simulink model "Sim_2025_04_07_Heet"  (R2024b)
settings: Solver=FixedStepAuto  StartTime=0.0  StopTime=2350  FixedStep=0.01  RelTol=1e-3
values from neighbouring files (symbols this model uses):
  cpSn = 230    [Sim_Parameter_Heet.m]
  mB = VB*rohSn    (= 7671.14496)    [Sim_Parameter_Heet.m]
  TU = 35    [Sim_Parameter_Heet.m]
undefined symbols (not defined in the file or in its folder): PLC_1, SIMATIC, UA
libraries: simulink x7, slpidlib x7, opcualib x6
(part 3 of 3)

== matlab function Sim_2025_04_07_Heet/Alte Systeme/Subsystem3/Air knife Betriebszustandsberechnung in Prozent ==
  data: druck1 input; druck2 input; Prozent output
function Prozent  = fcn(druck1, druck2)
%#codegen
% fcn Berechnet die Leistung und den prozentualen Anteil mithilfe einer
%     natürlichen Logarithmusfunktion.
%
% Eingänge:
%   druck1 - Erster Druckwert in mbar
%   druck2 - Zweiter Druckwert in mbar
%
% Ausgänge:
%   Leistung - Berechnete Leistung in Watt
%   Prozent  - Relativer Anteil in Prozent (0% - 100%)
%
% Randbedingungen:
%   - 0 mbar => 0%
%   - 400 mbar => 100%
%   - Dazwischen natürliche Logarithmus-Skalierung

    % Mittelwert berechnen
    druckMittelwert = (druck1 + druck2) / 2;
    
    % Sicherheitsabfragen, um log(0) zu vermeiden
    if druckMittelwert < 20
        druckMittelwert = 0;
    elseif druckMittelwert > 600
        druckMittelwert = 600;
    end

    
    if druckMittelwert == 0
        Prozent = 0;
    else
        Prozent = 100 *druckMittelwert / 600;
    end

    Leistung = (Prozent / 100) * 25900;
end

== matlab function Sim_2025_04_07_Heet/Aktuelle Systeme/Subsystem/MATLAB Function ==
  data: Bandnummer input; Dichte output; Cp20 output; Cp400 output
function [Dichte, Cp20, Cp400] = materialdaten(Bandnummer)
    % Materialdaten Tabelle
    Nr = (1:18)';

    % Dichte in kg/m³ (Umrechnung von g/cm³: * 1000)
    DichteList = [8960; 8960; 8900; 8850; 8800; 8800; 8800; 8800; 8750; 8750; 8900; 8900; 8900; 8800; 8800; 8900; 8900; 8200];

    % Thermische Leitfähigkeit bei 20°C in W/(m K)
    T_Leitfaeh20CList = [385; 385; 84; 82; 75; 75; 62; 62; 50; 120; 300; 260; 245; 190; 161; 197; 161; 81];

    % Thermische Leitfähigkeit bei 270°C in W/(m K)
    T_Leitfaeh270CList = [375; 375; 67; 35; 60; 60; 49; 49; 40; 103; 288; 214; 207; 160; 140; 175; 140; 68];

    % Wärmeausdehnungskoeffizient β in 1/K
    WaermeausdehnungskoefList = [1.77E-05; 1.77E-05; 1.82E-05; 1.82E-05; 1.85E-05; 1.85E-05; 1.85E-05; 1.85E-05; 1.84E-05; 1.84E-05; 1.80E-05; 1.68E-05; 1.68E-05; 1.70E-05; 1.70E-05; 1.70E-05; 1.70E-05; 1.82E-05];

    % Spezifische Wärmekapazität cp in J/(kg K) bei 20°C, 200°C, 400°C
    Cp20List = [385; 385; 360; 350; 340; 340; 330; 325; 320; 330; 385; 380; 375; 360; 365; 360; 355; 350];

    Cp200List = [388; 388; 370; 360; 360; 360; 340; 335; 340; 340; 388; 385; 380; 370; 375; 370; 365; 360];

    Cp400List = [391; 391; 380; 370; 370; 370; 350; 345; 350; 350; 391; 390; 385; 380; 380; 375; 370; 370];
    
    % Initialisierung der Ausgänge
    Dichte = 0;
    T_Leitfaeh20C = 0;
    T_Leitfaeh270C = 0;
    Waermeausdehnungskoef = 0;
    Cp20 = 0;
    Cp200 = 0;
    Cp400 = 0;

    % Prüfen, ob die Bandnummer gültig ist
    if Bandnummer > 0 && Bandnummer <= length(Nr)
        Dichte = DichteList(Bandnummer);
        T_Leitfaeh20C = T_Leitfaeh20CList(Bandnummer);
        T_Leitfaeh270C = T_Leitfaeh270CList(Bandnummer);
        Waermeausdehnungskoef = WaermeausdehnungskoefList(Bandnummer);
        Cp20 = Cp20List(Bandnummer);
        Cp200 = Cp200List(Bandnummer);
        Cp400 = Cp400List(Bandnummer);
    end
end

== matlab function Sim_2025_04_07_Heet/Alte Systeme/Subsystem3/Wärmestrom durch Band/MATLAB Function ==
  data: Bandnummer input; Dichte output; Cp20 output; Cp400 output
function [Dichte, Cp20, Cp400] = materialdaten(Bandnummer)
    % Materialdaten Tabelle
    Nr = (1:18)';

    % Dichte in kg/m³ (Umrechnung von g/cm³: * 1000)
    DichteList = [8960; 8960; 8900; 8850; 8800; 8800; 8800; 8800; 8750; 8750; 8900; 8900; 8900; 8800; 8800; 8900; 8900; 8200];

    % Thermische Leitfähigkeit bei 20°C in W/(m K)
    T_Leitfaeh20CList = [385; 385; 84; 82; 75; 75; 62; 62; 50; 120; 300; 260; 245; 190; 161; 197; 161; 81];

    % Thermische Leitfähigkeit bei 270°C in W/(m K)
    T_Leitfaeh270CList = [375; 375; 67; 35; 60; 60; 49; 49; 40; 103; 288; 214; 207; 160; 140; 175; 140; 68];

    % Wärmeausdehnungskoeffizient β in 1/K
    WaermeausdehnungskoefList = [1.77E-05; 1.77E-05; 1.82E-05; 1.82E-05; 1.85E-05; 1.85E-05; 1.85E-05; 1.85E-05; 1.84E-05; 1.84E-05; 1.80E-05; 1.68E-05; 1.68E-05; 1.70E-05; 1.70E-05; 1.70E-05; 1.70E-05; 1.82E-05];

    % Spezifische Wärmekapazität cp in J/(kg K) bei 20°C, 200°C, 400°C
    Cp20List = [385; 385; 360; 350; 340; 340; 330; 325; 320; 330; 385; 380; 375; 360; 365; 360; 355; 350];

    Cp200List = [388; 388; 370; 360; 360; 360; 340; 335; 340; 340; 388; 385; 380; 370; 375; 370; 365; 360];

    Cp400List = [391; 391; 380; 370; 370; 370; 350; 345; 350; 350; 391; 390; 385; 380; 380; 375; 370; 370];
    
    % Initialisierung der Ausgänge
    Dichte = 0;
    T_Leitfaeh20C = 0;
    T_Leitfaeh270C = 0;
    Waermeausdehnungskoef = 0;
    Cp20 = 0;
    Cp200 = 0;
    Cp400 = 0;

    % Prüfen, ob die Bandnummer gültig ist
    if Bandnummer > 0 && Bandnummer <= length(Nr)
        Dichte = DichteList(Bandnummer);
        T_Leitfaeh20C = T_Leitfaeh20CList(Bandnummer);
        T_Leitfaeh270C = T_Leitfaeh270CList(Bandnummer);
        Waermeausdehnungskoef = WaermeausdehnungskoefList(Bandnummer);
        Cp20 = Cp20List(Bandnummer);
        Cp200 = Cp200List(Bandnummer);
        Cp400 = Cp400List(Bandnummer);
    end
end

== matlab function Sim_2025_04_07_Heet/Alte Systeme/Subsystem3/Wärmestrom durch Band/MATLAB Function1 ==
  data: cp_20 input; cp_m output; cp_400 input; TU input; TuR input
function cp_m = cp_abhaengig_T(cp_20, cp_400, TU, TuR)
% Funktion zur Berechnung der Wärmekapazität bei der mittleren Temperatur

    % Mittlere Temperatur berechnen
    Tm = (TU + TuR) / 2;

    % Lineare Interpolation der Wärmekapazität
    % Annahme: Wärmekapazität ändert sich linear zwischen 20°C und 400°C
    cp_m = cp_20 + (cp_400 - cp_20) * (Tm - 20) / (400 - 20);

end

== matlab function Sim_2025_04_07_Heet/Alte Systeme/Subsystem4/Air knife Betriebszustandsberechnung in Prozent ==
  data: druck1 input; druck2 input; Prozent output
function Prozent  = fcn(druck1, druck2)
%#codegen
% fcn Berechnet die Leistung und den prozentualen Anteil mithilfe einer
%     natürlichen Logarithmusfunktion.
%
% Eingänge:
%   druck1 - Erster Druckwert in mbar
%   druck2 - Zweiter Druckwert in mbar
%
% Ausgänge:
%   Leistung - Berechnete Leistung in Watt
%   Prozent  - Relativer Anteil in Prozent (0% - 100%)
%
% Randbedingungen:
%   - 0 mbar => 0%
%   - 400 mbar => 100%
%   - Dazwischen natürliche Logarithmus-Skalierung

    % Mittelwert berechnen
    druckMittelwert = (druck1 + druck2) / 2;
    
    % Sicherheitsabfragen, um log(0) zu vermeiden
    if druckMittelwert < 20
        druckMittelwert = 0;
    elseif druckMittelwert > 600
        druckMittelwert = 600;
    end

    
    if druckMittelwert == 0
        Prozent = 0;
    else
        Prozent = 100 *druckMittelwert / 600;
    end

    Leistung = (Prozent / 100) * 25900;
end

== matlab function Sim_2025_04_07_Heet/Alte Systeme/Subsystem4/Wärmestrom durch Band/MATLAB Function ==
  data: Bandnummer input; Dichte output; Cp20 output; Cp400 output
function [Dichte, Cp20, Cp400] = materialdaten(Bandnummer)
    % Materialdaten Tabelle
    Nr = (1:18)';

    % Dichte in kg/m³ (Umrechnung von g/cm³: * 1000)
    DichteList = [8960; 8960; 8900; 8850; 8800; 8800; 8800; 8800; 8750; 8750; 8900; 8900; 8900; 8800; 8800; 8900; 8900; 8200];

    % Thermische Leitfähigkeit bei 20°C in W/(m K)
    T_Leitfaeh20CList = [385; 385; 84; 82; 75; 75; 62; 62; 50; 120; 300; 260; 245; 190; 161; 197; 161; 81];

    % Thermische Leitfähigkeit bei 270°C in W/(m K)
    T_Leitfaeh270CList = [375; 375; 67; 35; 60; 60; 49; 49; 40; 103; 288; 214; 207; 160; 140; 175; 140; 68];

    % Wärmeausdehnungskoeffizient β in 1/K
    WaermeausdehnungskoefList = [1.77E-05; 1.77E-05; 1.82E-05; 1.82E-05; 1.85E-05; 1.85E-05; 1.85E-05; 1.85E-05; 1.84E-05; 1.84E-05; 1.80E-05; 1.68E-05; 1.68E-05; 1.70E-05; 1.70E-05; 1.70E-05; 1.70E-05; 1.82E-05];

    % Spezifische Wärmekapazität cp in J/(kg K) bei 20°C, 200°C, 400°C
    Cp20List = [385; 385; 360; 350; 340; 340; 330; 325; 320; 330; 385; 380; 375; 360; 365; 360; 355; 350];

    Cp200List = [388; 388; 370; 360; 360; 360; 340; 335; 340; 340; 388; 385; 380; 370; 375; 370; 365; 360];

    Cp400List = [391; 391; 380; 370; 370; 370; 350; 345; 350; 350; 391; 390; 385; 380; 380; 375; 370; 370];
    
    % Initialisierung der Ausgänge
    Dichte = 0;
    T_Leitfaeh20C = 0;
    T_Leitfaeh270C = 0;
    Waermeausdehnungskoef = 0;
    Cp20 = 0;
    Cp200 = 0;
    Cp400 = 0;

    % Prüfen, ob die Bandnummer gültig ist
    if Bandnummer > 0 && Bandnummer <= length(Nr)
        Dichte = DichteList(Bandnummer);
        T_Leitfaeh20C = T_Leitfaeh20CList(Bandnummer);
        T_Leitfaeh270C = T_Leitfaeh270CList(Bandnummer);
        Waermeausdehnungskoef = WaermeausdehnungskoefList(Bandnummer);
        Cp20 = Cp20List(Bandnummer);
        Cp200 = Cp200List(Bandnummer);
        Cp400 = Cp400List(Bandnummer);
    end
end

== matlab function Sim_2025_04_07_Heet/Alte Systeme/Subsystem4/Wärmestrom durch Band/MATLAB Function1 ==
  data: cp_20 input; cp_m output; cp_400 input; TU input; TuR input
function cp_m = cp_abhaengig_T(cp_20, cp_400, TU, TuR)
% Funktion zur Berechnung der Wärmekapazität bei der mittleren Temperatur

    % Mittlere Temperatur berechnen
    Tm = (TU + TuR) / 2;

    % Lineare Interpolation der Wärmekapazität
    % Annahme: Wärmekapazität ändert sich linear zwischen 20°C und 400°C
    cp_m = cp_20 + (cp_400 - cp_20) * (Tm - 20) / (400 - 20);

end

== matlab function Sim_2025_04_07_Heet/Aktuelle Systeme/System mit Echtdatensätze/Air knife Betriebszustandsberechnung in Prozent ==
  data: druck1 input; druck2 input; Prozent output
function Prozent  = fcn(druck1, druck2)
%#codegen
% fcn Berechnet die Leistung und den prozentualen Anteil mithilfe einer
%     natürlichen Logarithmusfunktion.
%
% Eingänge:
%   druck1 - Erster Druckwert in mbar
%   druck2 - Zweiter Druckwert in mbar
%
% Ausgänge:
%   Leistung - Berechnete Leistung in Watt
%   Prozent  - Relativer Anteil in Prozent (0% - 100%)
%
% Randbedingungen:
%   - 0 mbar => 0%
%   - 400 mbar => 100%
%   - Dazwischen natürliche Logarithmus-Skalierung

    % Mittelwert berechnen
    druckMittelwert = (druck1 + druck2) / 2;
    
    % Sicherheitsabfragen, um log(0) zu vermeiden
    if druckMittelwert < 20
        druckMittelwert = 0;
    elseif druckMittelwert > 600
        druckMittelwert = 600;
    end

    
    if druckMittelwert == 0
        Prozent = 0;
    else
        Prozent = 100 *druckMittelwert / 600;
    end

    Leistung = (Prozent / 100) * 25900;
end

== matlab function Sim_2025_04_07_Heet/Aktuelle Systeme/System mit Echtdatensätze/MATLAB Function ==
  data: Zustand_Bandlauf input; y output; Solltemp_Stillstand input; Solltemp_Betrieb input
function y = fcn(Zustand_Bandlauf, Solltemp_Stillstand, Solltemp_Betrieb)
%#codegen
% Diese Funktion gibt abhängig vom Zustand_Bandlauf
% entweder die Solltemperatur im Stillstand oder im Betrieb aus.

    if Zustand_Bandlauf < 1
        y = Solltemp_Stillstand;
    else
        y = Solltemp_Betrieb;
    end
end

== matlab function Sim_2025_04_07_Heet/Aktuelle Systeme/System mit Echtdatensätze/MATLAB Function1 ==
  data: heizleistung input; korrHeiz output; zustand input; bandlaenge input
function korrHeiz = korrHeizleistung(heizleistung, zustand, bandlaenge)
%#codegen
% korrHeizleistung
%   Eingänge:
%       heizleistung: gewünschte Heizleistung [0…1] (z.B. 0.75 = 75%)
%       zustand:      0 oder 1
%       bandlaenge:   aktuelle Bandlänge
%
%   Ausgang:
%       korrHeiz:     korrigierte Heizleistung [0…1]

    if (zustand == 0) || (bandlaenge < 50)
        % Falls Zustand = 0 oder Bandlänge < 50,
        % wird die Heizleistung maximal auf 20 % (0.2) begrenzt.
        korrHeiz = min(heizleistung, 0.2);
    else
        % Ansonsten: gewünschte Heizleistung direkt durchreichen
        korrHeiz = heizleistung;
    end
end

== matlab function Sim_2025_04_07_Heet/Aktuelle Systeme/System mit Echtdatensätze/Wärmestrom durch Band/MATLAB Function ==
  data: Bandnummer input; Dichte output; Cp20 output; Cp400 output
function [Dichte, Cp20, Cp400] = materialdaten(Bandnummer)
    % Materialdaten Tabelle
    Nr = (1:18)';

    % Dichte in kg/m³ (Umrechnung von g/cm³: * 1000)
    DichteList = [8960; 8960; 8900; 8850; 8800; 8800; 8800; 8800; 8750; 8750; 8900; 8900; 8900; 8800; 8800; 8900; 8900; 8200];

    % Thermische Leitfähigkeit bei 20°C in W/(m K)
    T_Leitfaeh20CList = [385; 385; 84; 82; 75; 75; 62; 62; 50; 120; 300; 260; 245; 190; 161; 197; 161; 81];

    % Thermische Leitfähigkeit bei 270°C in W/(m K)
    T_Leitfaeh270CList = [375; 375; 67; 35; 60; 60; 49; 49; 40; 103; 288; 214; 207; 160; 140; 175; 140; 68];

    % Wärmeausdehnungskoeffizient β in 1/K
    WaermeausdehnungskoefList = [1.77E-05; 1.77E-05; 1.82E-05; 1.82E-05; 1.85E-05; 1.85E-05; 1.85E-05; 1.85E-05; 1.84E-05; 1.84E-05; 1.80E-05; 1.68E-05; 1.68E-05; 1.70E-05; 1.70E-05; 1.70E-05; 1.70E-05; 1.82E-05];

    % Spezifische Wärmekapazität cp in J/(kg K) bei 20°C, 200°C, 400°C
    Cp20List = [385; 385; 360; 350; 340; 340; 330; 325; 320; 330; 385; 380; 375; 360; 365; 360; 355; 350];

    Cp200List = [388; 388; 370; 360; 360; 360; 340; 335; 340; 340; 388; 385; 380; 370; 375; 370; 365; 360];

    Cp400List = [391; 391; 380; 370; 370; 370; 350; 345; 350; 350; 391; 390; 385; 380; 380; 375; 370; 370];
    
    % Initialisierung der Ausgänge
    Dichte = 0;
    T_Leitfaeh20C = 0;
    T_Leitfaeh270C = 0;
    Waermeausdehnungskoef = 0;
    Cp20 = 0;
    Cp200 = 0;
    Cp400 = 0;

    % Prüfen, ob die Bandnummer gültig ist
    if Bandnummer > 0 && Bandnummer <= length(Nr)
        Dichte = DichteList(Bandnummer);
        T_Leitfaeh20C = T_Leitfaeh20CList(Bandnummer);
        T_Leitfaeh270C = T_Leitfaeh270CList(Bandnummer);
        Waermeausdehnungskoef = WaermeausdehnungskoefList(Bandnummer);
        Cp20 = Cp20List(Bandnummer);
        Cp200 = Cp200List(Bandnummer);
        Cp400 = Cp400List(Bandnummer);
    end
end

== matlab function Sim_2025_04_07_Heet/Aktuelle Systeme/System mit Echtdatensätze/Wärmestrom durch Band/MATLAB Function1 ==
  data: cp_20 input; cp_m output; cp_400 input; TU input; TuR input
function cp_m = cp_abhaengig_T(cp_20, cp_400, TU, TuR)
% Funktion zur Berechnung der Wärmekapazität bei der mittleren Temperatur

    % Mittlere Temperatur berechnen
    Tm = (TU + TuR) / 2;

    % Lineare Interpolation der Wärmekapazität
    % Annahme: Wärmekapazität ändert sich linear zwischen 20°C und 400°C
    cp_m = cp_20 + (cp_400 - cp_20) * (Tm - 20) / (400 - 20);

end

== matlab function Sim_2025_04_07_Heet/Aktuelle Systeme/Subsystem/MATLAB Function1 ==
  data: cp_20 input; cp_m output; cp_400 input; TU input; TuR input
function cp_m = cp_abhaengig_T(cp_20, cp_400, TU, TuR)
% Funktion zur Berechnung der Wärmekapazität bei der mittleren Temperatur

    % Mittlere Temperatur berechnen
    Tm = (TU + TuR) / 2;

    % Lineare Interpolation der Wärmekapazität
    % Annahme: Wärmekapazität ändert sich linear zwischen 20°C und 400°C
    cp_m = cp_20 + (cp_400 - cp_20) * (Tm - 20) / (400 - 20);

end

== matlab function Sim_2025_04_07_Heet/Alte Systeme/Subsystem1/Air knife Betriebszustandsberechnung in Prozent ==
  data: druck1 input; druck2 input; Prozent output
function Prozent  = fcn(druck1, druck2)
%#codegen
% fcn Berechnet die Leistung und den prozentualen Anteil mithilfe einer
%     natürlichen Logarithmusfunktion.
%
% Eingänge:
%   druck1 - Erster Druckwert in mbar
%   druck2 - Zweiter Druckwert in mbar
%
% Ausgänge:
%   Leistung - Berechnete Leistung in Watt
%   Prozent  - Relativer Anteil in Prozent (0% - 100%)
%
% Randbedingungen:
%   - 0 mbar => 0%
%   - 400 mbar => 100%
%   - Dazwischen natürliche Logarithmus-Skalierung

    % Mittelwert berechnen
    druckMittelwert = (druck1 + druck2) / 2;
    
    % Sicherheitsabfragen, um log(0) zu vermeiden
    if druckMittelwert < 20
        druckMittelwert = 0;
    elseif druckMittelwert > 600
        druckMittelwert = 600;
    end

    
    if druckMittelwert == 0
        Prozent = 0;
    else
        Prozent = 100 *druckMittelwert / 600;
    end

    Leistung = (Prozent / 100) * 25900;
end

== matlab function Sim_2025_04_07_Heet/Alte Systeme/Subsystem1/Wärmestrom durch Band/MATLAB Function ==
  data: Bandnummer input; Dichte output; Cp20 output; Cp400 output
function [Dichte, Cp20, Cp400] = materialdaten(Bandnummer)
    % Materialdaten Tabelle
    Nr = (1:18)';

    % Dichte in kg/m³ (Umrechnung von g/cm³: * 1000)
    DichteList = [8960; 8960; 8900; 8850; 8800; 8800; 8800; 8800; 8750; 8750; 8900; 8900; 8900; 8800; 8800; 8900; 8900; 8200];

    % Thermische Leitfähigkeit bei 20°C in W/(m K)
    T_Leitfaeh20CList = [385; 385; 84; 82; 75; 75; 62; 62; 50; 120; 300; 260; 245; 190; 161; 197; 161; 81];

    % Thermische Leitfähigkeit bei 270°C in W/(m K)
    T_Leitfaeh270CList = [375; 375; 67; 35; 60; 60; 49; 49; 40; 103; 288; 214; 207; 160; 140; 175; 140; 68];

    % Wärmeausdehnungskoeffizient β in 1/K
    WaermeausdehnungskoefList = [1.77E-05; 1.77E-05; 1.82E-05; 1.82E-05; 1.85E-05; 1.85E-05; 1.85E-05; 1.85E-05; 1.84E-05; 1.84E-05; 1.80E-05; 1.68E-05; 1.68E-05; 1.70E-05; 1.70E-05; 1.70E-05; 1.70E-05; 1.82E-05];

    % Spezifische Wärmekapazität cp in J/(kg K) bei 20°C, 200°C, 400°C
    Cp20List = [385; 385; 360; 350; 340; 340; 330; 325; 320; 330; 385; 380; 375; 360; 365; 360; 355; 350];

    Cp200List = [388; 388; 370; 360; 360; 360; 340; 335; 340; 340; 388; 385; 380; 370; 375; 370; 365; 360];

    Cp400List = [391; 391; 380; 370; 370; 370; 350; 345; 350; 350; 391; 390; 385; 380; 380; 375; 370; 370];
    
    % Initialisierung der Ausgänge
    Dichte = 0;
    T_Leitfaeh20C = 0;
    T_Leitfaeh270C = 0;
    Waermeausdehnungskoef = 0;
    Cp20 = 0;
    Cp200 = 0;
    Cp400 = 0;

    % Prüfen, ob die Bandnummer gültig ist
    if Bandnummer > 0 && Bandnummer <= length(Nr)
        Dichte = DichteList(Bandnummer);
        T_Leitfaeh20C = T_Leitfaeh20CList(Bandnummer);
        T_Leitfaeh270C = T_Leitfaeh270CList(Bandnummer);
        Waermeausdehnungskoef = WaermeausdehnungskoefList(Bandnummer);
        Cp20 = Cp20List(Bandnummer);
        Cp200 = Cp200List(Bandnummer);
        Cp400 = Cp400List(Bandnummer);
    end
end

== matlab function Sim_2025_04_07_Heet/Aktuelle Systeme/System ohne Echtdatensätze/Air knife Betriebszustandsberechnung in Prozent ==
  data: druck1 input; druck2 input; Prozent output
function Prozent  = fcn(druck1, druck2)
%#codegen
% fcn Berechnet die Leistung und den prozentualen Anteil mithilfe einer
%     natürlichen Logarithmusfunktion.
%
% Eingänge:
%   druck1 - Erster Druckwert in mbar
%   druck2 - Zweiter Druckwert in mbar
%
% Ausgänge:
%   Leistung - Berechnete Leistung in Watt
%   Prozent  - Relativer Anteil in Prozent (0% - 100%)
%
% Randbedingungen:
%   - 0 mbar => 0%
%   - 400 mbar => 100%
%   - Dazwischen natürliche Logarithmus-Skalierung

    % Mittelwert berechnen
    druckMittelwert = (druck1 + druck2) / 2;
    
    % Sicherheitsabfragen, um log(0) zu vermeiden
    if druckMittelwert < 20
        druckMittelwert = 0;
    elseif druckMittelwert > 600
        druckMittelwert = 600;
    end

    
    if druckMittelwert == 0
        Prozent = 0;
    else
        Prozent = 100 *druckMittelwert / 600;
    end

    Leistung = (Prozent / 100) * 25900;
end

== matlab function Sim_2025_04_07_Heet/Aktuelle Systeme/System für Stillstand für Siemens/Wärmestrom durch Band/MATLAB Function ==
  data: Bandnummer input; Dichte output; Cp20 output; Cp400 output
function [Dichte, Cp20, Cp400] = materialdaten(Bandnummer)
    % Materialdaten Tabelle
    Nr = (1:18)';

    % Dichte in kg/m³ (Umrechnung von g/cm³: * 1000)
    DichteList = [8960; 8960; 8900; 8850; 8800; 8800; 8800; 8800; 8750; 8750; 8900; 8900; 8900; 8800; 8800; 8900; 8900; 8200];

    % Thermische Leitfähigkeit bei 20°C in W/(m K)
    T_Leitfaeh20CList = [385; 385; 84; 82; 75; 75; 62; 62; 50; 120; 300; 260; 245; 190; 161; 197; 161; 81];

    % Thermische Leitfähigkeit bei 270°C in W/(m K)
    T_Leitfaeh270CList = [375; 375; 67; 35; 60; 60; 49; 49; 40; 103; 288; 214; 207; 160; 140; 175; 140; 68];

    % Wärmeausdehnungskoeffizient β in 1/K
    WaermeausdehnungskoefList = [1.77E-05; 1.77E-05; 1.82E-05; 1.82E-05; 1.85E-05; 1.85E-05; 1.85E-05; 1.85E-05; 1.84E-05; 1.84E-05; 1.80E-05; 1.68E-05; 1.68E-05; 1.70E-05; 1.70E-05; 1.70E-05; 1.70E-05; 1.82E-05];

    % Spezifische Wärmekapazität cp in J/(kg K) bei 20°C, 200°C, 400°C
    Cp20List = [385; 385; 360; 350; 340; 340; 330; 325; 320; 330; 385; 380; 375; 360; 365; 360; 355; 350];

    Cp200List = [388; 388; 370; 360; 360; 360; 340; 335; 340; 340; 388; 385; 380; 370; 375; 370; 365; 360];

    Cp400List = [391; 391; 380; 370; 370; 370; 350; 345; 350; 350; 391; 390; 385; 380; 380; 375; 370; 370];
    
    % Initialisierung der Ausgänge
    Dichte = 0;
    T_Leitfaeh20C = 0;
    T_Leitfaeh270C = 0;
    Waermeausdehnungskoef = 0;
    Cp20 = 0;
    Cp200 = 0;
    Cp400 = 0;

    % Prüfen, ob die Bandnummer gültig ist
    if Bandnummer > 0 && Bandnummer <= length(Nr)
        Dichte = DichteList(Bandnummer);
        T_Leitfaeh20C = T_Leitfaeh20CList(Bandnummer);
        T_Leitfaeh270C = T_Leitfaeh270CList(Bandnummer);
        Waermeausdehnungskoef = WaermeausdehnungskoefList(Bandnummer);
        Cp20 = Cp20List(Bandnummer);
        Cp200 = Cp200List(Bandnummer);
        Cp400 = Cp400List(Bandnummer);
    end
end

== matlab function Sim_2025_04_07_Heet/Aktuelle Systeme/System für Stillstand für Siemens/Wärmestrom durch Band/MATLAB Function1 ==
  data: cp_20 input; cp_m output; cp_400 input; TU input; TuR input
function cp_m = cp_abhaengig_T(cp_20, cp_400, TU, TuR)
% Funktion zur Berechnung der Wärmekapazität bei der mittleren Temperatur

    % Mittlere Temperatur berechnen
    Tm = (TU + TuR) / 2;

    % Lineare Interpolation der Wärmekapazität
    % Annahme: Wärmekapazität ändert sich linear zwischen 20°C und 400°C
    cp_m = cp_20 + (cp_400 - cp_20) * (Tm - 20) / (400 - 20);

end

== matlab function Sim_2025_04_07_Heet/Aktuelle Systeme/System ohne Echtdatensätze/Wärmestrom durch Band/MATLAB Function ==
  data: Bandnummer input; Dichte output; Cp20 output; Cp400 output
function [Dichte, Cp20, Cp400] = materialdaten(Bandnummer)
    % Materialdaten Tabelle
    Nr = (1:18)';

    % Dichte in kg/m³ (Umrechnung von g/cm³: * 1000)
    DichteList = [8960; 8960; 8900; 8850; 8800; 8800; 8800; 8800; 8750; 8750; 8900; 8900; 8900; 8800; 8800; 8900; 8900; 8200];

    % Thermische Leitfähigkeit bei 20°C in W/(m K)
    T_Leitfaeh20CList = [385; 385; 84; 82; 75; 75; 62; 62; 50; 120; 300; 260; 245; 190; 161; 197; 161; 81];

    % Thermische Leitfähigkeit bei 270°C in W/(m K)
    T_Leitfaeh270CList = [375; 375; 67; 35; 60; 60; 49; 49; 40; 103; 288; 214; 207; 160; 140; 175; 140; 68];

    % Wärmeausdehnungskoeffizient β in 1/K
    WaermeausdehnungskoefList = [1.77E-05; 1.77E-05; 1.82E-05; 1.82E-05; 1.85E-05; 1.85E-05; 1.85E-05; 1.85E-05; 1.84E-05; 1.84E-05; 1.80E-05; 1.68E-05; 1.68E-05; 1.70E-05; 1.70E-05; 1.70E-05; 1.70E-05; 1.82E-05];

    % Spezifische Wärmekapazität cp in J/(kg K) bei 20°C, 200°C, 400°C
    Cp20List = [385; 385; 360; 350; 340; 340; 330; 325; 320; 330; 385; 380; 375; 360; 365; 360; 355; 350];

    Cp200List = [388; 388; 370; 360; 360; 360; 340; 335; 340; 340; 388; 385; 380; 370; 375; 370; 365; 360];

    Cp400List = [391; 391; 380; 370; 370; 370; 350; 345; 350; 350; 391; 390; 385; 380; 380; 375; 370; 370];
    
    % Initialisierung der Ausgänge
    Dichte = 0;
    T_Leitfaeh20C = 0;
    T_Leitfaeh270C = 0;
    Waermeausdehnungskoef = 0;
    Cp20 = 0;
    Cp200 = 0;
    Cp400 = 0;

    % Prüfen, ob die Bandnummer gültig ist
    if Bandnummer > 0 && Bandnummer <= length(Nr)
        Dichte = DichteList(Bandnummer);
        T_Leitfaeh20C = T_Leitfaeh20CList(Bandnummer);
        T_Leitfaeh270C = T_Leitfaeh270CList(Bandnummer);
        Waermeausdehnungskoef = WaermeausdehnungskoefList(Bandnummer);
        Cp20 = Cp20List(Bandnummer);
        Cp200 = Cp200List(Bandnummer);
        Cp400 = Cp400List(Bandnummer);
    end
end

== matlab function Sim_2025_04_07_Heet/Aktuelle Systeme/System ohne Echtdatensätze/Wärmestrom durch Band/MATLAB Function1 ==
  data: cp_20 input; cp_m output; cp_400 input; TU input; TuR input
function cp_m = cp_abhaengig_T(cp_20, cp_400, TU, TuR)
% Funktion zur Berechnung der Wärmekapazität bei der mittleren Temperatur

    % Mittlere Temperatur berechnen
    Tm = (TU + TuR) / 2;

    % Lineare Interpolation der Wärmekapazität
    % Annahme: Wärmekapazität ändert sich linear zwischen 20°C und 400°C
    cp_m = cp_20 + (cp_400 - cp_20) * (Tm - 20) / (400 - 20);

end

== matlab function Sim_2025_04_07_Heet/Alte Systeme/Subsystem1/Wärmestrom durch Band/MATLAB Function1 ==
  data: cp_20 input; cp_m output; cp_400 input; TU input; TuR input
function cp_m = cp_abhaengig_T(cp_20, cp_400, TU, TuR)
% Funktion zur Berechnung der Wärmekapazität bei der mittleren Temperatur

    % Mittlere Temperatur berechnen
    Tm = (TU + TuR) / 2;

    % Lineare Interpolation der Wärmekapazität
    % Annahme: Wärmekapazität ändert sich linear zwischen 20°C und 400°C
    cp_m = cp_20 + (cp_400 - cp_20) * (Tm - 20) / (400 - 20);

end
